simulink model "Simscape_task2_motors"  (R2024b)
settings: Solver=FixedStepAuto  StartTime=0.0  StopTime=t_all(end)  FixedStep=0.001  RelTol=1e-3
values from neighbouring files (symbols this model uses):
  l0 = 200e-3    (= 0.2)    [LinesParabolas_task1.m]    (also in PlotArea4R_Catalog.m = L(1); PlotRobot2.m = L(1); PlotRobot3.m = L(1); ROBOTdir_4R.m = L(1))
  l1 = 329e-3    (= 0.329)    [LinesParabolas_task1.m]    (also in PlotArea4R_Catalog.m = L(2); PlotRobot2.m = L(2); PlotRobot3.m = L(2); ROBOTdir_4R.m = L(2))
  l2 = 311.50e-3    (= 0.3115)    [LinesParabolas_task1.m]    (also in PlotArea4R_Catalog.m = L(3); PlotRobot2.m = L(3); PlotRobot3.m = L(3); ROBOTdir_4R.m = L(3))
  l3 = 106e-3    (= 0.106)    [LinesParabolas_task1.m]    (also in PlotArea4R_Catalog.m = L(4); PlotRobot2.m = L(4); PlotRobot3.m = L(4); ROBOTdir_4R.m = L(4))
  m0 = 17    [LinesParabolas_task1.m]    (also in Sshape_task2.m)
  m1 = 10    [LinesParabolas_task1.m]    (also in Sshape_task2.m)
  m2 = 9    [LinesParabolas_task1.m]    (also in Sshape_task2.m)
  m3 = 3    [LinesParabolas_task1.m]    (also in Sshape_task2.m)
  N = length(t_all)    [LinesParabolas_task1.m]
  q_all = zeros(4, N)    [LinesParabolas_task1.m]    (also in Sshape_task2.m = zeros(nJ, Nt))
  rid = 1/100    (= 0.01)    [LinesParabolas_task1.m]    (also in Sshape_task2.m)
  s = svd(Jv)    [LinesParabolas_task1.m]    (also in Sshape_task2.m; test_robot_4R_Conditioning.m)
  X = [250 270 300 340 370 420 500 420 370 340 300 250 ] * 1e-3    [LinesParabolas_task1.m]    (also in PlotArea4R_Catalog.m = X(idx); test_robot_4R_Conditioning.m = X(idx))
  Y = zeros(size(X))    [LinesParabolas_task1.m]    (also in PlotArea4R_Catalog.m = Y(idx); test_robot_4R_Conditioning.m = Y(idx))
  Z = [ 75 75 75 150 180 220 230 220 180 150 75 75 ] * 1e-3    [LinesParabolas_task1.m]    (also in PlotArea4R_Catalog.m = Z(idx); test_robot_4R_Conditioning.m = Z(idx))
libraries: fl_lib x52, nesl_utility x34, sm_lib x24, SignalEditorBlockLib x4
(part 2 of 2)

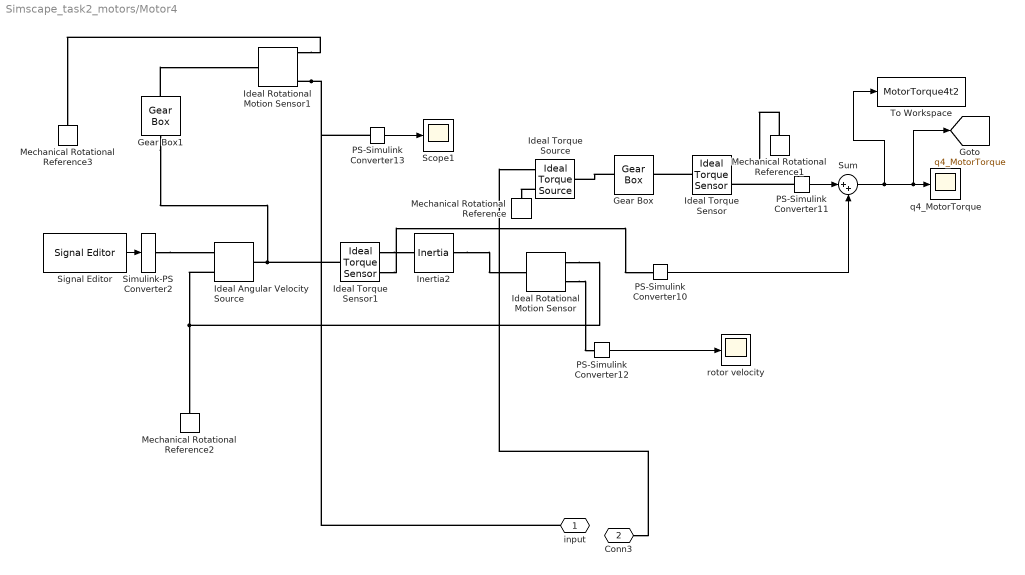
== system Simscape_task2_motors/Motor4 ==
  Gear Box : fl_lib/Mechanical/Mechanisms/Gear Box  ratio=rid  t_in_specify=off  t_in_priority=None  t_in=0 N*m  t_in_nominal_specify=off  t_in_nominal_value=1  t_in_nominal_unit=N*m  t_out_specify=off  t_out_priority=None  t_out=0 N*m  t_out_nominal_specify=off  t_out_nominal_value=1  t_out_nominal_unit=N*m
  Gear Box1 : fl_lib/Mechanical/Mechanisms/Gear Box  ratio=1/rid  t_in_specify=off  t_in_priority=None  t_in=0 N*m  t_in_nominal_specify=off  t_in_nominal_value=1  t_in_nominal_unit=N*m  t_out_specify=off  t_out_priority=None  t_out=0 N*m  t_out_nominal_specify=off  t_out_nominal_value=1  t_out_nominal_unit=N*m
  Ideal Angular Velocity Source : fl_lib/Mechanical/Mechanical Sources/Ideal Angular Velocity Source
  Ideal Rotational Motion Sensor : fl_lib/Mechanical/Mechanical Sensors/Ideal Rotational Motion Sensor  reference=foundation.enum.MeasurementReference.difference  acceleration_port=false  velocity_port=true  position_port=false  wrap_angle=false  offset=0 rad
      settings: InternalSimscapePortConfiguration="{\"Bottom\":[],\"Left\":[{\"id\":\"R\",\"label\":\"R\",\"type\":\"foundation.mechanical.rotational.rotational\"}],\"Right\":[{\"id\":\"C\",\"label\":\"C\",\"type\":\"foundation.mechanical.rotational.rotational\"},{\"id\":\"W\",\"label\":\"W\",\"type\":\"output\"}],\"Top\":[]}"
  Ideal Rotational Motion Sensor1 : fl_lib/Mechanical/Mechanical Sensors/Ideal Rotational Motion Sensor  reference=foundation.enum.MeasurementReference.difference  acceleration_port=false  velocity_port=true  position_port=true  wrap_angle=false  offset=q_all(4,1) rad
  Ideal Torque Sensor : fl_lib/Mechanical/Mechanical Sensors/Ideal Torque Sensor
  Ideal Torque Sensor1 : fl_lib/Mechanical/Mechanical Sensors/Ideal Torque Sensor
  Ideal Torque Source : fl_lib/Mechanical/Mechanical Sources/Ideal Torque Source
  Inertia2 : fl_lib/Mechanical/Rotational Elements/Inertia  inertia=mot_inertia kg*m^2  num_ports=foundation.enum.numPorts2.two  w_specify=off  w_priority=High  w=209 rad/s  w_nominal_specify=off  w_nominal_value=209  w_nominal_unit=rad/s  t_specify=off  t_priority=None  t=0 N*m  t_nominal_specify=off  t_nominal_value=1  t_nominal_unit=N*m
      settings: InternalSimscapePortConfiguration="{\"Bottom\":[],\"Left\":[{\"id\":\"I\",\"label\":\"\",\"type\":\"foundation.mechanical.rotational.rotational\"}],\"Right\":[{\"id\":\"J\",\"label\":\"\",\"type\":\"foundation.mechanical.rotational.rotational\"}],\"Top\":[]}"
  Mechanical Rotational Reference{,1..3} (4 alike) : fl_lib/Mechanical/Rotational Elements/Mechanical Rotational Reference
  PS-Simulink Converter{10..13} (4 alike) : nesl_utility/PS-Simulink Converter  PhysicalDomain=network_engine_domain  SubClassName=ps_output  LeftPortType=input  RightPortType=output  PseudoPeriodic=off  Frequencies=[]  VectorFormat=inherit  Unit=inherit  AffineConversion=off
  Scope1 : Scope
  Signal Editor : SignalEditorBlockLib/Signal Editor  FileName=vel4_task2.mat  ActiveScenario=ds4_task2  ActiveSignal=velocity  IsBus=off  OutputBusObjectStr=Bus: BusObject  SampleTime=0  Interpolate=off  ZeroCross=off  OutputAfterFinalValue=Setting to zero  Unit=inherit  PreserveSignalName=on  ApplySigPropsToAllScenarios=on  ApplySigPropsToAllSignals=off
  Simulink-PS Converter2 : nesl_utility/Simulink-PS Converter  PhysicalDomain=network_engine_domain  SubClassName=ps_input  LeftPortType=input  RightPortType=output  PseudoPeriodic=off  Frequencies=[]  NoiseDistribution=none  NoiseParameters=[]  Unit=rad/s  AffineConversion=off  FilteringAndDerivatives=filter  SimscapeFilterOrder=2  InputFilterTimeConstant=0.001  UdotUserProvided=2
  Sum : Sum  Inputs=|++
  To Workspace : ToWorkspace  VariableName=MotorTorque4t2  SaveFormat=Timeseries  SampleTime=-1
  q4_MotorTorque : Scope
  rotor velocity : Scope
  input : PMIOPort  Side=Right
  Conn3 : PMIOPort  Port=2  Side=Right
  tag scope: q4_MotorTorque=global
  wires:
  PS-Simulink Converter12/1 -> rotor velocity/1
  PS-Simulink Converter10/1 -> Sum/2
  PS-Simulink Converter13/1 -> Scope1/1
  Sum/1 -> To Workspace/1, [q4_MotorTorque], q4_MotorTorque/1
  PS-Simulink Converter11/1 -> Sum/1
  Signal Editor/1 -> Simulink-PS Converter2/1
  connections:
  Ideal Rotational Motion Sensor1/RConn3 -- PS-Simulink Converter13/LConn1 -- input/RConn1
  PS-Simulink Converter11/LConn1 -- Ideal Torque Sensor/RConn2
  Ideal Torque Sensor/LConn1 -- Gear Box/RConn1
  Ideal Rotational Motion Sensor/RConn2 -- PS-Simulink Converter12/LConn1
  Ideal Torque Sensor1/RConn1 -- Inertia2/RConn1
  Mechanical Rotational Reference1/LConn1 -- Ideal Torque Sensor/RConn1
  Inertia2/LConn1 -- Ideal Rotational Motion Sensor/LConn1
  Ideal Torque Source/RConn2 -- Mechanical Rotational Reference/LConn1
  Gear Box1/RConn1 -- Ideal Rotational Motion Sensor1/LConn1
  Simulink-PS Converter2/RConn1 -- Ideal Angular Velocity Source/RConn1
  Ideal Torque Sensor1/RConn2 -- PS-Simulink Converter10/LConn1
  Ideal Rotational Motion Sensor/RConn1 -- Mechanical Rotational Reference2/LConn1 -- Ideal Angular Velocity Source/RConn2
  Conn3/RConn1 -- Ideal Torque Source/RConn1
  Ideal Rotational Motion Sensor1/RConn1 -- Mechanical Rotational Reference3/LConn1
  Ideal Torque Sensor1/LConn1 -- Ideal Angular Velocity Source/LConn1 -- Gear Box1/LConn1
  Gear Box/LConn1 -- Ideal Torque Source/LConn1
